simulink model "Project_Earth_Pointing"  (R2022b)
settings: Solver=VariableStepAuto  StartTime=0.0  StopTime=1000  RelTol=1e-3
values from neighbouring files (symbols this model uses):
  a = (Rp+Ra)/2    [trial_complete_project.m]    (also in trial_detumbling.m; trial_earth_pointing.m)
  A0 = Ax*Ay*Az    [trial_complete_project.m]    (also in trial_detumbling.m = [0.5391 0.1008 0.8362; -0.3591 0.9255 0.1200; -0.7618 -0.365; trial_earth_pointing.m = [-0.2505 -0.7848 0.5668; 0.7978 0.1644 0.5801; -0.5485 0.597)
  A1 = L1*L2    (= 0.06)    [trial_complete_project.m]    (also in trial_detumbling.m; trial_earth_pointing.m)
  A10 = A1    (= 0.06)    [trial_complete_project.m]    (also in trial_detumbling.m; trial_earth_pointing.m)
  A2 = A1    (= 0.06)    [trial_complete_project.m]    (also in trial_detumbling.m; trial_earth_pointing.m)
  A3 = L1*L3    (= 0.03)    [trial_complete_project.m]    (also in trial_detumbling.m; trial_earth_pointing.m)
  A4 = A3    (= 0.03)    [trial_complete_project.m]    (also in trial_detumbling.m; trial_earth_pointing.m)
  A5 = L2*L3    (= 0.02)    [trial_complete_project.m]    (also in trial_detumbling.m; trial_earth_pointing.m)
  A6 = A5    (= 0.02)    [trial_complete_project.m]    (also in trial_detumbling.m; trial_earth_pointing.m)
  A7 = A1    (= 0.06)    [trial_complete_project.m]    (also in trial_detumbling.m; trial_earth_pointing.m)
  A8 = A1    (= 0.06)    [trial_complete_project.m]    (also in trial_detumbling.m; trial_earth_pointing.m)
  A9 = A1    (= 0.06)    [trial_complete_project.m]    (also in trial_detumbling.m; trial_earth_pointing.m)
  a_s = 149600000    [trial_complete_project.m]    (also in trial_detumbling.m; trial_earth_pointing.m)
  alpha1 = 0.9    [trial_complete_project.m]    (also in trial_detumbling.m; trial_earth_pointing.m)
  alpha2 = 0.1    [trial_complete_project.m]    (also in trial_detumbling.m; trial_earth_pointing.m)
  alphaState_obs = -0.9    [trial_complete_project.m]    (also in trial_detumbling.m; trial_earth_pointing.m)
  an = (11.5*pi)/180    (= 0.200712863979)    [trial_complete_project.m]    (also in trial_detumbling.m; trial_earth_pointing.m)
  e = (Ra-Rp)/(Ra+Rp)    [trial_complete_project.m]    (also in trial_detumbling.m; trial_earth_pointing.m)
  e_s = 0.0167086    [trial_complete_project.m]    (also in trial_detumbling.m; trial_earth_pointing.m)
  i = 0*pi/180    (= 0)    [trial_complete_project.m]    (also in trial_detumbling.m; trial_earth_pointing.m)
  I_x = 0.059029338    [trial_complete_project.m]    (also in trial_detumbling.m; trial_earth_pointing.m = 0.093296)
  I_y = 0.116709338    [trial_complete_project.m]    (also in trial_detumbling.m; trial_earth_pointing.m = 0.161261916)
  I_z = 0.149968    [trial_complete_project.m]    (also in trial_detumbling.m; trial_earth_pointing.m = 0.160253916)
  kdx = kd*(I_x/I)    (= 1.44987726319)    [trial_complete_project.m]    (also in trial_detumbling.m; trial_earth_pointing.m = 2.6989394073)
  kdy = kd*(I_y/I)    (= 2.86661211697)    [trial_complete_project.m]    (also in trial_detumbling.m; trial_earth_pointing.m = 4.66511040119)
  kdz = kd*(I_z/I)    (= 3.68351061984)    [trial_complete_project.m]    (also in trial_detumbling.m; trial_earth_pointing.m = 4.63595019151)
  kpx = kp*(I_x/I)    (= 0.0163111192108)    [trial_complete_project.m]    (also in trial_detumbling.m; trial_earth_pointing.m = 0.0202420455548)
  kpy = kp*(I_y/I)    (= 0.0322493863159)    [trial_complete_project.m]    (also in trial_detumbling.m; trial_earth_pointing.m = 0.0349883280089)
  kpz = kp*(I_z/I)    (= 0.0414394944732)    [trial_complete_project.m]    (also in trial_detumbling.m; trial_earth_pointing.m = 0.0347696264363)
  kState_obs = 0.9    [trial_complete_project.m]    (also in trial_detumbling.m; trial_earth_pointing.m)
  m = [0.01 0.05 0.01]    [trial_complete_project.m]    (also in trial_detumbling.m; trial_earth_pointing.m)
  mu = astroConstants(13)    [trial_complete_project.m]    (also in trial_detumbling.m; trial_earth_pointing.m)
  n = sqrt(mu/a^3)    [trial_complete_project.m]    (also in trial_detumbling.m; trial_earth_pointing.m)
  n_s = sqrt(mu_s/a_s^3)    [trial_complete_project.m]    (also in trial_detumbling.m; trial_earth_pointing.m)
  P = F_e/c    (= 4.52980041279e-06)    [trial_complete_project.m]    (also in trial_detumbling.m; trial_earth_pointing.m)
  P_E = F_earth/c    (= 2.23487943783e-06)    [trial_complete_project.m]    (also in trial_detumbling.m; trial_earth_pointing.m)
  pd_sc = 0.1    [trial_complete_project.m]    (also in trial_detumbling.m; trial_earth_pointing.m)
  pd_sp = 0.1    [trial_complete_project.m]    (also in trial_detumbling.m; trial_earth_pointing.m)
  ps_sc = 0.5    [trial_complete_project.m]    (also in trial_detumbling.m; trial_earth_pointing.m)
  ps_sp = 0.1    [trial_complete_project.m]    (also in trial_detumbling.m; trial_earth_pointing.m)
  r = astroConstants(23)    [trial_complete_project.m]    (also in trial_detumbling.m; trial_earth_pointing.m)
  r1 = [0;0;-L3/2] + c_m    [trial_complete_project.m]    (also in trial_detumbling.m; trial_earth_pointing.m)
  r10 = r9    [trial_complete_project.m]    (also in trial_detumbling.m; trial_earth_pointing.m)
  r2 = [0; 0 ;L3/2] + c_m    [trial_complete_project.m]    (also in trial_detumbling.m; trial_earth_pointing.m)
  r3 = [0; L2/2;0] + c_m    [trial_complete_project.m]    (also in trial_detumbling.m; trial_earth_pointing.m)
  r4 = [0; -L2/2;0] + c_m    [trial_complete_project.m]    (also in trial_detumbling.m; trial_earth_pointing.m)
  r5 = [-L1/2; 0 ;0] + c_m    [trial_complete_project.m]    (also in trial_detumbling.m; trial_earth_pointing.m)
  r6 = [L1/2; 0;0]+ c_m    [trial_complete_project.m]    (also in trial_detumbling.m; trial_earth_pointing.m)
  r7 = [-L1/2; 0 ; L3/2 + L1/2] + c_m    [trial_complete_project.m]    (also in trial_detumbling.m; trial_earth_pointing.m)
  r8 = r7    [trial_complete_project.m]    (also in trial_detumbling.m; trial_earth_pointing.m)
  r9 = [-L1/2; 0 ; -L3/2 - L1/2]    [trial_complete_project.m]    (also in trial_detumbling.m; trial_earth_pointing.m)
  RW = 0.002    [trial_complete_project.m]    (also in trial_detumbling.m; trial_earth_pointing.m)
  theta0 = 0    [trial_complete_project.m]    (also in trial_detumbling.m; trial_earth_pointing.m)
  w0_x = 1    [trial_complete_project.m]    (also in trial_detumbling.m; trial_earth_pointing.m = -0.008328)
  w0_y = 1    [trial_complete_project.m]    (also in trial_detumbling.m; trial_earth_pointing.m = 0.004962)
  w0_z = 1    [trial_complete_project.m]    (also in trial_detumbling.m; trial_earth_pointing.m = -0.0004756)
  w_E = (15.04*pi/180)/3600    (= 7.29159776389e-05)    [trial_complete_project.m]    (also in trial_detumbling.m; trial_earth_pointing.m)
libraries: matrix_library x28, vrlib x7, dspinverses x1
(part 3 of 3)

== system Project_Earth_Pointing/Environment/SRP Torque/Subsystem5 ==
  Input : Inport
  Input1 : Inport  Port=2
  Constant : Constant
  Constant1 : Constant  Value=ps_sc
  Constant2 : Constant  Value=pd_sc
  Dot Product : DotProduct  OutDataTypeStr=Inherit: Inherit via internal rule
  Gain : Gain  Gain=-P
  Gain1 : Gain  Gain=A5
  Gain2 : Gain  Gain=2
  Gain3 : Gain  Gain=2/3
  Product{,1..3} (4 alike) : Product
  Sum : Sum  Inputs=|+-
  Sum1 : Sum  Inputs=|++
  Sum2 : Sum  Inputs=|++
  Output : Outport
  Output1 : Outport  Port=2
  wires:
  Input1/1 -> Dot Product/2, Product3/2  "N_B"
  Product2/1 -> Sum2/1
  Product1/1 -> Sum1/1
  Constant2/1 -> Gain3/1
  Sum/1 -> Product1/1
  Constant1/1 -> Gain2/1, Sum/2
  Sum1/1 -> Product/2
  Product/1 -> Output/1
  Dot Product/1 -> Output1/1, Product2/2, Gain/1
  Gain/1 -> Gain1/1
  Gain1/1 -> Product/1
  Sum2/1 -> Product3/1
  Input/1 -> Product1/2, Dot Product/1  "S-B"
  Gain2/1 -> Product2/1
  Constant/1 -> Sum/1
  Product3/1 -> Sum1/2
  Gain3/1 -> Sum2/2

== system Project_Earth_Pointing/Environment/SRP Torque/Subsystem6 ==
  Input : Inport
  Input1 : Inport  Port=2
  Constant : Constant
  Constant1 : Constant  Value=ps_sc
  Constant2 : Constant  Value=pd_sc
  Dot Product : DotProduct  OutDataTypeStr=Inherit: Inherit via internal rule
  Gain : Gain  Gain=-P
  Gain1 : Gain  Gain=A6
  Gain2 : Gain  Gain=2
  Gain3 : Gain  Gain=2/3
  Product{,1..3} (4 alike) : Product
  Sum : Sum  Inputs=|+-
  Sum1 : Sum  Inputs=|++
  Sum2 : Sum  Inputs=|++
  Output : Outport
  Output1 : Outport  Port=2
  wires:
  Gain3/1 -> Sum2/2
  Product3/1 -> Sum1/2
  Constant/1 -> Sum/1
  Gain2/1 -> Product2/1
  Input/1 -> Dot Product/1, Product1/2  "S-B"
  Sum2/1 -> Product3/1
  Gain1/1 -> Product/1
  Gain/1 -> Gain1/1
  Dot Product/1 -> Gain/1, Product2/2, Output1/1
  Product/1 -> Output/1
  Sum1/1 -> Product/2
  Constant1/1 -> Sum/2, Gain2/1
  Sum/1 -> Product1/1
  Constant2/1 -> Gain3/1
  Product1/1 -> Sum1/1
  Product2/1 -> Sum2/1
  Input1/1 -> Product3/2, Dot Product/2  "N_B"

== system Project_Earth_Pointing/Environment/SRP Torque/Subsystem7 ==
  Input : Inport
  Input1 : Inport  Port=2
  Constant : Constant
  Constant1 : Constant  Value=ps_sp
  Constant2 : Constant  Value=pd_sp
  Dot Product : DotProduct  OutDataTypeStr=Inherit: Inherit via internal rule
  Gain : Gain  Gain=-P
  Gain1 : Gain  Gain=A7
  Gain2 : Gain  Gain=2
  Gain3 : Gain  Gain=2/3
  Product{,1..3} (4 alike) : Product
  Sum : Sum  Inputs=|+-
  Sum1 : Sum  Inputs=|++
  Sum2 : Sum  Inputs=|++
  Output : Outport
  Output1 : Outport  Port=2
  wires:
  Input1/1 -> Dot Product/2, Product3/2  "N_B"
  Product2/1 -> Sum2/1
  Product1/1 -> Sum1/1
  Constant2/1 -> Gain3/1
  Sum/1 -> Product1/1
  Constant1/1 -> Gain2/1, Sum/2
  Sum1/1 -> Product/2
  Product/1 -> Output/1
  Dot Product/1 -> Output1/1, Product2/2, Gain/1
  Gain/1 -> Gain1/1
  Gain1/1 -> Product/1
  Sum2/1 -> Product3/1
  Input/1 -> Product1/2, Dot Product/1  "S-B"
  Gain2/1 -> Product2/1
  Constant/1 -> Sum/1
  Product3/1 -> Sum1/2
  Gain3/1 -> Sum2/2

== system Project_Earth_Pointing/Environment/SRP Torque/Subsystem8 ==
  Input : Inport
  Input1 : Inport  Port=2
  Constant : Constant
  Constant1 : Constant  Value=ps_sp
  Constant2 : Constant  Value=pd_sp
  Dot Product : DotProduct  OutDataTypeStr=Inherit: Inherit via internal rule
  Gain : Gain  Gain=-P
  Gain1 : Gain  Gain=A8
  Gain2 : Gain  Gain=2
  Gain3 : Gain  Gain=2/3
  Product{,1..3} (4 alike) : Product
  Sum : Sum  Inputs=|+-
  Sum1 : Sum  Inputs=|++
  Sum2 : Sum  Inputs=|++
  Output : Outport
  Output1 : Outport  Port=2
  wires:
  Gain3/1 -> Sum2/2
  Product3/1 -> Sum1/2
  Constant/1 -> Sum/1
  Gain2/1 -> Product2/1
  Input/1 -> Dot Product/1, Product1/2  "S-B"
  Sum2/1 -> Product3/1
  Gain1/1 -> Product/1
  Gain/1 -> Gain1/1
  Dot Product/1 -> Gain/1, Product2/2, Output1/1
  Product/1 -> Output/1
  Sum1/1 -> Product/2
  Constant1/1 -> Sum/2, Gain2/1
  Sum/1 -> Product1/1
  Constant2/1 -> Gain3/1
  Product1/1 -> Sum1/1
  Product2/1 -> Sum2/1
  Input1/1 -> Product3/2, Dot Product/2  "N_B"

== system Project_Earth_Pointing/Environment/SRP Torque/Subsystem9 ==
  Input : Inport
  Input1 : Inport  Port=2
  Constant : Constant
  Constant1 : Constant  Value=ps_sp
  Constant2 : Constant  Value=pd_sp
  Dot Product : DotProduct  OutDataTypeStr=Inherit: Inherit via internal rule
  Gain : Gain  Gain=-P
  Gain1 : Gain  Gain=A9
  Gain2 : Gain  Gain=2
  Gain3 : Gain  Gain=2/3
  Product{,1..3} (4 alike) : Product
  Sum : Sum  Inputs=|+-
  Sum1 : Sum  Inputs=|++
  Sum2 : Sum  Inputs=|++
  Output : Outport
  Output1 : Outport  Port=2
  wires:
  Input1/1 -> Dot Product/2, Product3/2  "N_B"
  Product2/1 -> Sum2/1
  Product1/1 -> Sum1/1
  Constant2/1 -> Gain3/1
  Sum/1 -> Product1/1
  Constant1/1 -> Gain2/1, Sum/2
  Sum1/1 -> Product/2
  Product/1 -> Output/1
  Dot Product/1 -> Output1/1, Product2/2, Gain/1
  Gain/1 -> Gain1/1
  Gain1/1 -> Product/1
  Sum2/1 -> Product3/1
  Input/1 -> Product1/2, Dot Product/1  "S-B"
  Gain2/1 -> Product2/1
  Constant/1 -> Sum/1
  Product3/1 -> Sum1/2
  Gain3/1 -> Sum2/2

== system Project_Earth_Pointing/Environment/SRP Torque/Theta_integration ==
  Constant : Constant
  Constant1 : Constant  Value=e
  Constant2 : Constant  Value=e
  Constant3 : Constant
  Constant4 : Constant  Value=3/2
  Cos : Trigonometry  Operator=cos
  Divide : Product  Inputs=*/
  Gain : Gain  Gain=n
  Integrator : Integrator  InitialCondition=theta0
  Product : Product
  Scope : Scope
  Square : Math  Operator=square
  Square1 : Math  Operator=square
  Square2 : Math  Operator=pow
  Sum : Sum  Inputs=|++
  Sum1 : Sum  Inputs=|+-
  Output : Outport
  wires:
  Gain/1 -> Divide/1
  Constant4/1 -> Square2/2
  Square2/1 -> Divide/2
  Sum/1 -> Square/1
  Divide/1 -> Integrator/1
  Square/1 -> Gain/1
  Constant2/1 -> Square1/1
  Sum1/1 -> Square2/1
  Constant/1 -> Sum/2
  Square1/1 -> Sum1/2
  Product/1 -> Sum/1
  Cos/1 -> Product/2
  Constant3/1 -> Sum1/1
  Integrator/1 -> Cos/1, Scope/1, Output/1
  Constant1/1 -> Product/1

== system Project_Earth_Pointing/Reaction Wheel/If Action Subsystem/If Action Subsystem ==
  Action Port : ActionPort  ActionPortLabel=if(u1 <RWmin)
  Constant : Constant  Value=0
  Out1 : Outport
  wires:
  Constant/1 -> Out1/1

== system Project_Earth_Pointing/Reaction Wheel/If Action Subsystem/If Action Subsystem1 ==
  Action Port : ActionPort  ActionPortLabel=elseif(u1>=RW)
  Constant : Constant  Value=RW
  Out1 : Outport
  wires:
  Constant/1 -> Out1/1

== system Project_Earth_Pointing/Reaction Wheel/If Action Subsystem/If Action Subsystem2 ==
  Input : Inport
  Action Port : ActionPort  ActionPortLabel=else
  Out1 : Outport
  wires:
  Input/1 -> Out1/1

== system Project_Earth_Pointing/Reaction Wheel/If Action Subsystem1/If Action Subsystem ==
  Action Port : ActionPort  ActionPortLabel=if(u1 >-RWmin)
  Constant : Constant  Value=0
  Out1 : Outport
  wires:
  Constant/1 -> Out1/1

== system Project_Earth_Pointing/Reaction Wheel/If Action Subsystem1/If Action Subsystem1 ==
  Action Port : ActionPort  ActionPortLabel=elseif(u1<=-RW)
  Constant : Constant  Value=-RW
  Out1 : Outport
  wires:
  Constant/1 -> Out1/1

== system Project_Earth_Pointing/Reaction Wheel/If Action Subsystem1/If Action Subsystem2 ==
  Input : Inport
  Action Port : ActionPort  ActionPortLabel=else
  Out1 : Outport
  wires:
  Input/1 -> Out1/1

== system Project_Earth_Pointing/Reaction Wheel/If Action Subsystem2/If Action Subsystem ==
  Action Port : ActionPort  ActionPortLabel=if(u1 <RWmin)
  Constant : Constant  Value=0
  Out1 : Outport
  wires:
  Constant/1 -> Out1/1

== system Project_Earth_Pointing/Reaction Wheel/If Action Subsystem2/If Action Subsystem1 ==
  Action Port : ActionPort  ActionPortLabel=elseif(u1>=RW)
  Constant : Constant  Value=RW
  Out1 : Outport
  wires:
  Constant/1 -> Out1/1

== system Project_Earth_Pointing/Reaction Wheel/If Action Subsystem2/If Action Subsystem2 ==
  Input : Inport
  Action Port : ActionPort  ActionPortLabel=else
  Out1 : Outport
  wires:
  Input/1 -> Out1/1

== system Project_Earth_Pointing/Reaction Wheel/If Action Subsystem3/If Action Subsystem ==
  Action Port : ActionPort  ActionPortLabel=if(u1 >-RWmin)
  Constant : Constant  Value=0
  Out1 : Outport
  wires:
  Constant/1 -> Out1/1

== system Project_Earth_Pointing/Reaction Wheel/If Action Subsystem3/If Action Subsystem1 ==
  Action Port : ActionPort  ActionPortLabel=elseif(u1<=-RW)
  Constant : Constant  Value=-RW
  Out1 : Outport
  wires:
  Constant/1 -> Out1/1

== system Project_Earth_Pointing/Reaction Wheel/If Action Subsystem3/If Action Subsystem2 ==
  Input : Inport
  Action Port : ActionPort  ActionPortLabel=else
  Out1 : Outport
  wires:
  Input/1 -> Out1/1

== system Project_Earth_Pointing/Reaction Wheel/If Action Subsystem4/If Action Subsystem ==
  Action Port : ActionPort  ActionPortLabel=if(u1 <RWmin)
  Constant : Constant  Value=0
  Out1 : Outport
  wires:
  Constant/1 -> Out1/1

== system Project_Earth_Pointing/Reaction Wheel/If Action Subsystem4/If Action Subsystem1 ==
  Action Port : ActionPort  ActionPortLabel=elseif(u1>=RW)
  Constant : Constant  Value=RW
  Out1 : Outport
  wires:
  Constant/1 -> Out1/1

== system Project_Earth_Pointing/Reaction Wheel/If Action Subsystem4/If Action Subsystem2 ==
  Input : Inport
  Action Port : ActionPort  ActionPortLabel=else
  Out1 : Outport
  wires:
  Input/1 -> Out1/1

== system Project_Earth_Pointing/Reaction Wheel/If Action Subsystem5/If Action Subsystem ==
  Action Port : ActionPort  ActionPortLabel=if(u1 >-RWmin)
  Constant : Constant  Value=0
  Out1 : Outport
  wires:
  Constant/1 -> Out1/1

== system Project_Earth_Pointing/Reaction Wheel/If Action Subsystem5/If Action Subsystem1 ==
  Action Port : ActionPort  ActionPortLabel=elseif(u1<=-RW)
  Constant : Constant  Value=-RW
  Out1 : Outport
  wires:
  Constant/1 -> Out1/1

== system Project_Earth_Pointing/Reaction Wheel/If Action Subsystem5/If Action Subsystem2 ==
  Input : Inport
  Action Port : ActionPort  ActionPortLabel=else
  Out1 : Outport
  wires:
  Input/1 -> Out1/1

== system Project_Earth_Pointing/Environment/ERP Torque/Subsystem11/If Action Subsystem ==
  Action Port : ActionPort  ActionPortLabel=else
  Constant : Constant  Value=[0 0 0]'
  Out1 : Outport
  wires:
  Constant/1 -> Out1/1

== system Project_Earth_Pointing/Environment/ERP Torque/Subsystem11/If Action Subsystem1 ==
  Action Port : ActionPort  ActionPortLabel=else
  Constant : Constant  Value=[0 0 0]'
  Out1 : Outport
  wires:
  Constant/1 -> Out1/1

== system Project_Earth_Pointing/Environment/ERP Torque/Subsystem11/If Action Subsystem2 ==
  Action Port : ActionPort  ActionPortLabel=else
  Constant : Constant  Value=[0 0 0]'
  Out1 : Outport
  wires:
  Constant/1 -> Out1/1

== system Project_Earth_Pointing/Environment/ERP Torque/Subsystem11/If Action Subsystem3 ==
  Action Port : ActionPort  ActionPortLabel=else
  Constant : Constant  Value=[0 0 0]'
  Out1 : Outport
  wires:
  Constant/1 -> Out1/1

== system Project_Earth_Pointing/Environment/ERP Torque/Subsystem11/If Action Subsystem4 ==
  Action Port : ActionPort  ActionPortLabel=else
  Constant : Constant  Value=[0 0 0]'
  Out1 : Outport
  wires:
  Constant/1 -> Out1/1

== system Project_Earth_Pointing/Environment/ERP Torque/Subsystem11/If Action Subsystem5 ==
  Action Port : ActionPort  ActionPortLabel=else
  Constant : Constant  Value=[0 0 0]'
  Out1 : Outport
  wires:
  Constant/1 -> Out1/1

== system Project_Earth_Pointing/Environment/ERP Torque/Subsystem11/If Action Subsystem6 ==
  Action Port : ActionPort  ActionPortLabel=else
  Constant : Constant  Value=[0 0 0]'
  Out1 : Outport
  wires:
  Constant/1 -> Out1/1

== system Project_Earth_Pointing/Environment/ERP Torque/Subsystem11/If Action Subsystem7 ==
  Action Port : ActionPort  ActionPortLabel=else
  Constant : Constant  Value=[0 0 0]'
  Out1 : Outport
  wires:
  Constant/1 -> Out1/1

== system Project_Earth_Pointing/Environment/ERP Torque/Subsystem11/If Action Subsystem8 ==
  Action Port : ActionPort  ActionPortLabel=else
  Constant : Constant  Value=[0 0 0]'
  Out1 : Outport
  wires:
  Constant/1 -> Out1/1

== system Project_Earth_Pointing/Environment/ERP Torque/Subsystem11/If Action Subsystem9 ==
  Action Port : ActionPort  ActionPortLabel=else
  Constant : Constant  Value=[0 0 0]'
  Out1 : Outport
  wires:
  Constant/1 -> Out1/1

== system Project_Earth_Pointing/Environment/ERP Torque/Subsystem11/Subsystem ==
  Input3 : Inport
  Action Port : ActionPort  ActionPortLabel=if(u1 > 0)
  Constant : Constant  Value=r1
  Cross Product : matrix_library/Cross Product
  Output : Outport
  wires:
  Cross Product/1 -> Output/1
  Constant/1 -> Cross Product/1
  Input3/1 -> Cross Product/2

== system Project_Earth_Pointing/Environment/ERP Torque/Subsystem11/Subsystem1 ==
  Input3 : Inport
  Action Port : ActionPort  ActionPortLabel=if(u1 > 0)
  Constant : Constant  Value=r2
  Cross Product : matrix_library/Cross Product
  Output : Outport
  wires:
  Input3/1 -> Cross Product/2
  Constant/1 -> Cross Product/1
  Cross Product/1 -> Output/1

== system Project_Earth_Pointing/Environment/ERP Torque/Subsystem11/Subsystem2 ==
  Input3 : Inport
  Action Port : ActionPort  ActionPortLabel=if(u1 > 0)
  Constant : Constant  Value=r3
  Cross Product : matrix_library/Cross Product
  Output : Outport
  wires:
  Cross Product/1 -> Output/1
  Constant/1 -> Cross Product/1
  Input3/1 -> Cross Product/2

== system Project_Earth_Pointing/Environment/ERP Torque/Subsystem11/Subsystem3 ==
  Input3 : Inport
  Action Port : ActionPort  ActionPortLabel=if(u1 > 0)
  Constant : Constant  Value=r4
  Cross Product : matrix_library/Cross Product
  Output : Outport
  wires:
  Input3/1 -> Cross Product/2
  Constant/1 -> Cross Product/1
  Cross Product/1 -> Output/1

== system Project_Earth_Pointing/Environment/ERP Torque/Subsystem11/Subsystem4 ==
  Input3 : Inport
  Action Port : ActionPort  ActionPortLabel=if(u1 > 0)
  Constant : Constant  Value=r5
  Cross Product : matrix_library/Cross Product
  Output : Outport
  wires:
  Cross Product/1 -> Output/1
  Constant/1 -> Cross Product/1
  Input3/1 -> Cross Product/2

== system Project_Earth_Pointing/Environment/ERP Torque/Subsystem11/Subsystem5 ==
  Input3 : Inport
  Action Port : ActionPort  ActionPortLabel=if(u1 > 0)
  Constant : Constant  Value=r6
  Cross Product : matrix_library/Cross Product
  Output : Outport
  wires:
  Input3/1 -> Cross Product/2
  Constant/1 -> Cross Product/1
  Cross Product/1 -> Output/1

== system Project_Earth_Pointing/Environment/ERP Torque/Subsystem11/Subsystem6 ==
  Input3 : Inport
  Action Port : ActionPort  ActionPortLabel=if(u1 > 0)
  Constant : Constant  Value=r7
  Cross Product : matrix_library/Cross Product
  Output : Outport
  wires:
  Cross Product/1 -> Output/1
  Constant/1 -> Cross Product/1
  Input3/1 -> Cross Product/2

== system Project_Earth_Pointing/Environment/ERP Torque/Subsystem11/Subsystem7 ==
  Input3 : Inport
  Action Port : ActionPort  ActionPortLabel=if(u1 > 0)
  Constant : Constant  Value=r8
  Cross Product : matrix_library/Cross Product
  Output : Outport
  wires:
  Input3/1 -> Cross Product/2
  Constant/1 -> Cross Product/1
  Cross Product/1 -> Output/1

== system Project_Earth_Pointing/Environment/ERP Torque/Subsystem11/Subsystem8 ==
  Input3 : Inport
  Action Port : ActionPort  ActionPortLabel=if(u1 > 0)
  Constant : Constant  Value=r9
  Cross Product : matrix_library/Cross Product
  Display : Display
  Output : Outport
  wires:
  Cross Product/1 -> Output/1
  Constant/1 -> Cross Product/1
  Input3/1 -> Cross Product/2, Display/1

== system Project_Earth_Pointing/Environment/ERP Torque/Subsystem11/Subsystem9 ==
  Input3 : Inport
  Action Port : ActionPort  ActionPortLabel=if(u1 > 0)
  Constant : Constant  Value=r10
  Cross Product : matrix_library/Cross Product
  Output : Outport
  wires:
  Input3/1 -> Cross Product/2
  Constant/1 -> Cross Product/1
  Cross Product/1 -> Output/1

== system Project_Earth_Pointing/Environment/Gravity Torque/Two_body_problem/R ==
  Input : Inport
  Constant1 : Constant
  Constant2 : Constant  Value=e
  Constant3 : Constant
  Constant4 : Constant  Value=e
  Cos2 : Trigonometry  Operator=cos
  Divide : Product  Inputs=*/  RndMeth=Zero  SaturateOnIntegerOverflow=on
  Gain : Gain  Gain=a
  Product2 : Product
  Square : Math  Operator=square
  Sum : Sum  Inputs=|+-
  Sum1 : Sum  Inputs=|++
  Output : Outport
  wires:
  Sum1/1 -> Divide/2
  Product2/1 -> Sum1/2
  Constant4/1 -> Product2/1
  Constant3/1 -> Sum1/1
  Gain/1 -> Divide/1
  Sum/1 -> Gain/1
  Square/1 -> Sum/2
  Constant2/1 -> Square/1
  Constant1/1 -> Sum/1
  Input/1 -> Cos2/1
  Cos2/1 -> Product2/2
  Divide/1 -> Output/1

== system Project_Earth_Pointing/Environment/Gravity Torque/Two_body_problem/Theta_integration ==
  Constant : Constant
  Constant1 : Constant  Value=e
  Constant2 : Constant  Value=e
  Constant3 : Constant
  Constant4 : Constant  Value=3/2
  Cos : Trigonometry  Operator=cos
  Divide : Product  Inputs=*/
  Gain : Gain  Gain=n
  Integrator : Integrator  InitialCondition=theta0
  Product : Product
  Scope : Scope
  Square : Math  Operator=square
  Square1 : Math  Operator=square
  Square2 : Math  Operator=pow
  Sum : Sum  Inputs=|++
  Sum1 : Sum  Inputs=|+-
  Output : Outport
  wires:
  Constant1/1 -> Product/1
  Integrator/1 -> Output/1, Scope/1, Cos/1
  Constant3/1 -> Sum1/1
  Cos/1 -> Product/2
  Product/1 -> Sum/1
  Square1/1 -> Sum1/2
  Constant/1 -> Sum/2
  Sum1/1 -> Square2/1
  Constant2/1 -> Square1/1
  Square/1 -> Gain/1
  Divide/1 -> Integrator/1
  Sum/1 -> Square/1
  Square2/1 -> Divide/2
  Constant4/1 -> Square2/2
  Gain/1 -> Divide/1

== system Project_Earth_Pointing/Environment/SRP Torque/Subsystem11/If Action Subsystem ==
  Action Port : ActionPort  ActionPortLabel=else
  Constant : Constant  Value=[0 0 0]'
  Out1 : Outport
  wires:
  Constant/1 -> Out1/1

== system Project_Earth_Pointing/Environment/SRP Torque/Subsystem11/If Action Subsystem1 ==
  Action Port : ActionPort  ActionPortLabel=else
  Constant : Constant  Value=[0 0 0]'
  Out1 : Outport
  wires:
  Constant/1 -> Out1/1

== system Project_Earth_Pointing/Environment/SRP Torque/Subsystem11/If Action Subsystem2 ==
  Action Port : ActionPort  ActionPortLabel=else
  Constant : Constant  Value=[0 0 0]'
  Out1 : Outport
  wires:
  Constant/1 -> Out1/1

== system Project_Earth_Pointing/Environment/SRP Torque/Subsystem11/If Action Subsystem3 ==
  Action Port : ActionPort  ActionPortLabel=else
  Constant : Constant  Value=[0 0 0]'
  Out1 : Outport
  wires:
  Constant/1 -> Out1/1

== system Project_Earth_Pointing/Environment/SRP Torque/Subsystem11/If Action Subsystem4 ==
  Action Port : ActionPort  ActionPortLabel=else
  Constant : Constant  Value=[0 0 0]'
  Out1 : Outport
  wires:
  Constant/1 -> Out1/1

== system Project_Earth_Pointing/Environment/SRP Torque/Subsystem11/If Action Subsystem5 ==
  Action Port : ActionPort  ActionPortLabel=else
  Constant : Constant  Value=[0 0 0]'
  Out1 : Outport
  wires:
  Constant/1 -> Out1/1

== system Project_Earth_Pointing/Environment/SRP Torque/Subsystem11/If Action Subsystem6 ==
  Action Port : ActionPort  ActionPortLabel=else
  Constant : Constant  Value=[0 0 0]'
  Out1 : Outport
  wires:
  Constant/1 -> Out1/1

== system Project_Earth_Pointing/Environment/SRP Torque/Subsystem11/If Action Subsystem7 ==
  Action Port : ActionPort  ActionPortLabel=else
  Constant : Constant  Value=[0 0 0]'
  Out1 : Outport
  wires:
  Constant/1 -> Out1/1

== system Project_Earth_Pointing/Environment/SRP Torque/Subsystem11/If Action Subsystem8 ==
  Action Port : ActionPort  ActionPortLabel=else
  Constant : Constant  Value=[0 0 0]'
  Out1 : Outport
  wires:
  Constant/1 -> Out1/1

== system Project_Earth_Pointing/Environment/SRP Torque/Subsystem11/If Action Subsystem9 ==
  Action Port : ActionPort  ActionPortLabel=else
  Constant : Constant  Value=[0 0 0]'
  Out1 : Outport
  wires:
  Constant/1 -> Out1/1

== system Project_Earth_Pointing/Environment/SRP Torque/Subsystem11/Subsystem ==
  Input3 : Inport
  Action Port : ActionPort  ActionPortLabel=if(u1 > 0)
  Constant : Constant  Value=r1
  Cross Product : matrix_library/Cross Product
  Output : Outport
  wires:
  Input3/1 -> Cross Product/2
  Constant/1 -> Cross Product/1
  Cross Product/1 -> Output/1

== system Project_Earth_Pointing/Environment/SRP Torque/Subsystem11/Subsystem1 ==
  Input3 : Inport
  Action Port : ActionPort  ActionPortLabel=if(u1 > 0)
  Constant : Constant  Value=r2
  Cross Product : matrix_library/Cross Product
  Output : Outport
  wires:
  Cross Product/1 -> Output/1
  Constant/1 -> Cross Product/1
  Input3/1 -> Cross Product/2

== system Project_Earth_Pointing/Environment/SRP Torque/Subsystem11/Subsystem2 ==
  Input3 : Inport
  Action Port : ActionPort  ActionPortLabel=if(u1 > 0)
  Constant : Constant  Value=r3
  Cross Product : matrix_library/Cross Product
  Output : Outport
  wires:
  Input3/1 -> Cross Product/2
  Constant/1 -> Cross Product/1
  Cross Product/1 -> Output/1

== system Project_Earth_Pointing/Environment/SRP Torque/Subsystem11/Subsystem3 ==
  Input3 : Inport
  Action Port : ActionPort  ActionPortLabel=if(u1 > 0)
  Constant : Constant  Value=r4
  Cross Product : matrix_library/Cross Product
  Output : Outport
  wires:
  Cross Product/1 -> Output/1
  Constant/1 -> Cross Product/1
  Input3/1 -> Cross Product/2

== system Project_Earth_Pointing/Environment/SRP Torque/Subsystem11/Subsystem4 ==
  Input3 : Inport
  Action Port : ActionPort  ActionPortLabel=if(u1 > 0)
  Constant : Constant  Value=r5
  Cross Product : matrix_library/Cross Product
  Output : Outport
  wires:
  Input3/1 -> Cross Product/2
  Constant/1 -> Cross Product/1
  Cross Product/1 -> Output/1

== system Project_Earth_Pointing/Environment/SRP Torque/Subsystem11/Subsystem5 ==
  Input3 : Inport
  Action Port : ActionPort  ActionPortLabel=if(u1 > 0)
  Constant : Constant  Value=r6
  Cross Product : matrix_library/Cross Product
  Output : Outport
  wires:
  Cross Product/1 -> Output/1
  Constant/1 -> Cross Product/1
  Input3/1 -> Cross Product/2

== system Project_Earth_Pointing/Environment/SRP Torque/Subsystem11/Subsystem6 ==
  Input3 : Inport
  Action Port : ActionPort  ActionPortLabel=if(u1 > 0)
  Constant : Constant  Value=r7
  Cross Product : matrix_library/Cross Product
  Output : Outport
  wires:
  Input3/1 -> Cross Product/2
  Constant/1 -> Cross Product/1
  Cross Product/1 -> Output/1

== system Project_Earth_Pointing/Environment/SRP Torque/Subsystem11/Subsystem7 ==
  Input3 : Inport
  Action Port : ActionPort  ActionPortLabel=if(u1 > 0)
  Constant : Constant  Value=r8
  Cross Product : matrix_library/Cross Product
  Output : Outport
  wires:
  Cross Product/1 -> Output/1
  Constant/1 -> Cross Product/1
  Input3/1 -> Cross Product/2

== system Project_Earth_Pointing/Environment/SRP Torque/Subsystem11/Subsystem8 ==
  Input3 : Inport
  Action Port : ActionPort  ActionPortLabel=if(u1 > 0)
  Constant : Constant  Value=r9
  Cross Product : matrix_library/Cross Product
  Display : Display
  Output : Outport
  wires:
  Input3/1 -> Display/1, Cross Product/2
  Constant/1 -> Cross Product/1
  Cross Product/1 -> Output/1

== system Project_Earth_Pointing/Environment/SRP Torque/Subsystem11/Subsystem9 ==
  Input3 : Inport
  Action Port : ActionPort  ActionPortLabel=if(u1 > 0)
  Constant : Constant  Value=r10
  Cross Product : matrix_library/Cross Product
  Output : Outport
  wires:
  Cross Product/1 -> Output/1
  Constant/1 -> Cross Product/1
  Input3/1 -> Cross Product/2

== matlab function Project_Earth_Pointing/Attitude Determination/MATLAB Function ==
  data: B input; U output; M output; V output
function [U,M,V]  = fcn(B)

[U,S,V] = svd(B);

M=diag([1 1 det(U)*det(V)]);

end
